simulink model "Kontinuierlich_state"  (Simulink 9.1)
settings: Solver=ode15s  StartTime=0.0  StopTime=10  RelTol=1e-2  EnableMultiTasking=on
values from neighbouring files (symbols this model uses):
  b1 = 2.39e6    (= 2390000)    [main4.m]
  c_oe = 36.5e6    (= 36500000)    [main4.m]
  c_p = 75e6    (= 75000000)    [main4.m]
  m_g = m_k + m_p    (= 268.7)    [main4.m]
libraries: simulink x1
settings Model: Creator=yjl_9  LastModifiedBy=Emily
settings DataIOCC: LimitDataPoints=on
settings DebuggingCC: SolverPrmCheckMsg=warning
settings GRTTargetCC: GeneratePreprocessorConditionals=Disable all  CombineOutputUpdateFcns=on  GRTInterface=off

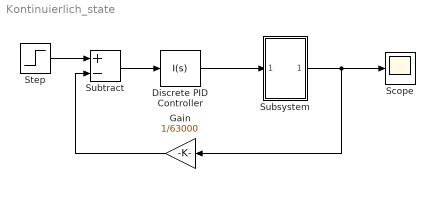
== system Kontinuierlich_state ==
  Discrete PID Controller : simulink/Continuous/PID Controller  Controller=I  TimeDomain=Continuous-time  SampleTime=-1  IntegratorMethod=Forward Euler  FilterMethod=Forward Euler  Form=Parallel  UseFilter=on  ControllerParametersSource=internal  P=0  I=0.25  D=0  N=100  InitialConditionSource=internal  InitialConditionForIntegrator=0  InitialConditionForFilter=0  ExternalReset=none  LimitOutput=off  UpperSaturationLimit=inf  LowerSaturationLimit=-inf  LinearizeAsGain=off  AntiWindupMode=none  Kb=1  TrackingMode=off  Kt=1  PParamMin=[]  PParamMax=[]  IParamMin=[]  IParamMax=[]  DParamMin=[]  DParamMax=[]  NParamMin=[]  NParamMax=[]  KbParamMin=[]  KbParamMax=[]  KtParamMin=[]  KtParamMax=[]  POutMin=[]  POutMax=[]  IOutMin=[]  IOutMax=[]  DOutMin=[]  DOutMax=[]  NOutMin=[]  NOutMax=[]  KbOutMin=[]  KbOutMax=[]  KtOutMin=[]  KtOutMax=[]  IntegratorOutMin=[]  IntegratorOutMax=[]  FilterOutMin=[]  FilterOutMax=[]  SumOutMin=[]  SumOutMax=[]  SumI1OutMin=[]  SumI1OutMax=[]  SumI2OutMin=[]  SumI2OutMax=[]  SumI3OutMin=[]  SumI3OutMax=[]  SumDOutMin=[]  SumDOutMax=[]  SaturationOutMin=[]  SaturationOutMax=[]  IntegratorContinuousStateAttributes=''  IntegratorStateMustResolveToSignalObject=off  IntegratorRTWStateStorageClass=Auto  FilterContinuousStateAttributes=''  FilterStateMustResolveToSignalObject=off  FilterRTWStateStorageClass=Auto  DifferentiatorICPrevScaledInput=0  DifferentiatorOutMin=[]  DifferentiatorOutMax=[]  FilterDiffOutCoefMin=[]  FilterDiffOutCoefMax=[]  SumDenOutMin=[]  SumDenOutMax=[]  SumNumOutMin=[]  SumNumOutMax=[]  ReciprocalOutMin=[]  ReciprocalOutMax=[]  DivideOutMin=[]  DivideOutMax=[]  TunerSelectOption=Transfer Function Based (PID Tuner App)
  Gain : Gain  Gain=1/63000
  Scope : Scope
  Step : Step  After=0.8
  Subsystem : Subsystem
  Subtract : Sum  Inputs=+-
  wires:
  Gain/1 -> Subtract/2
  Step/1 -> Subtract/1
  Subtract/1 -> Discrete PID Controller/1
  Subsystem/1(Out2) -> Gain/1, Scope/1
  Discrete PID Controller/1 -> Subsystem/1(In1)

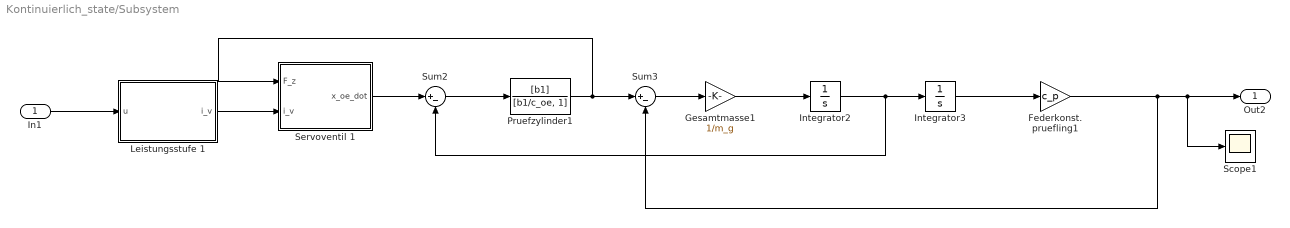
== system Kontinuierlich_state/Subsystem ==
  In1 : Inport
  Federkonst. pruefling1 : Gain  Gain=c_p
  Gesamtmasse1 : Gain  Gain=1/m_g
  Integrator2 : Integrator
  Integrator3 : Integrator
  Leistungsstufe 1 : MATLAB Function  TreatAsAtomicUnit=on
  Pruefzylinder1 : TransferFcn  Numerator=[b1]  Denominator=[b1/c_oe, 1]
  Scope1 : Scope
  Servoventil 1 : MATLAB Function  TreatAsAtomicUnit=on
  Sum2 : Sum  Inputs=|+-
  Sum3 : Sum  Inputs=|+-
  Out2 : Outport
  wires:
  Leistungsstufe 1/1(i_v) -> Servoventil 1/2(i_v)
  Servoventil 1/1(x_oe_dot) -> Sum2/1
  In1/1 -> Leistungsstufe 1/1(u)
  Integrator2/1 -> Sum2/2, Integrator3/1
  Federkonst. pruefling1/1 -> Sum3/2, Scope1/1, Out2/1
  Integrator3/1 -> Federkonst. pruefling1/1
  Sum2/1 -> Pruefzylinder1/1
  Sum3/1 -> Gesamtmasse1/1
  Gesamtmasse1/1 -> Integrator2/1
  Pruefzylinder1/1 -> Servoventil 1/1(F_z), Sum3/1

== matlab function Subsystem/Leistungsstufe 1 ==
  data: u input double; i_v output double
function i_v  = leistungsstufe(u)
%codegen
i_max = 1; % [A]
K_L = 1; % [A/V]
    if u > 1
        i_v = i_max;
    elseif u < -1
        i_v = -i_max;
    else 
        i_v = K_L*u;
    end

== matlab function Subsystem/Servoventil 1 ==
  data: F_z input double; i_v input double; x_oe_dot output double
function x_oe_dot = servoventil(F_z,i_v)
%#codegen
K_sv = 0.796; % [m/As]
F_N = 63000; % [N]
A = 1-(F_z/F_N)*sign(i_v);

if A > 0
    x_oe_dot = i_v*K_sv*sqrt(A);
else 
    x_oe_dot = 0;
end
